simulink model "esempio2S"  (R2020a)
settings: Solver=VariableStepAuto  StartTime=0.0  StopTime=10.0  RelTol=1e-3
values from neighbouring files (symbols this model uses):
  K = place(A, B, P)    [esempio.m]    (also in esempio1.m = acker(A, B, P); esempio2.m)
settings Model: Creator=itama  LastModifiedBy=itama

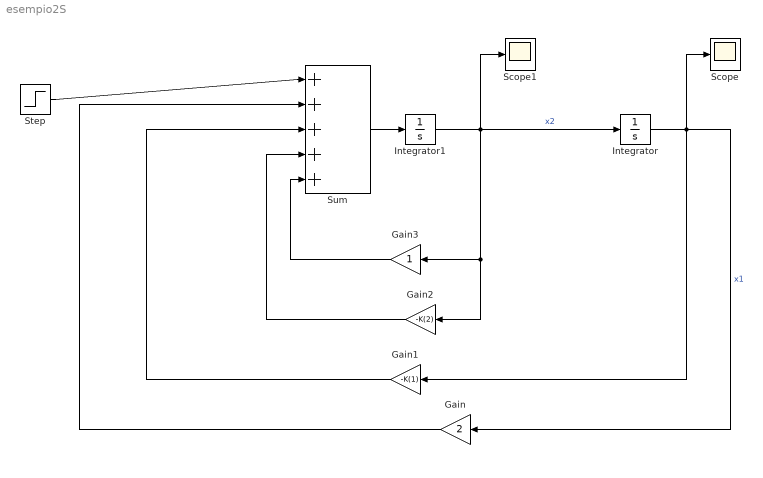
== system esempio2S ==
  Gain : Gain  Gain=2
  Gain1 : Gain  Gain=-K(1)
  Gain2 : Gain  Gain=-K(2)
  Gain3 : Gain
  Integrator : Integrator
  Integrator1 : Integrator
  Scope : Scope
  Scope1 : Scope
  Step : Step  SampleTime=0
  Sum : Sum  Inputs=|+++++
  wires:
  Integrator1/1 -> Gain3/1, Gain2/1, Scope1/1, Integrator/1  "x2"
  Integrator/1 -> Gain1/1, Gain/1, Scope/1  "x1"
  Step/1 -> Sum/1
  Sum/1 -> Integrator1/1
  Gain/1 -> Sum/2
  Gain3/1 -> Sum/5
  Gain2/1 -> Sum/4
  Gain1/1 -> Sum/3
